simulink model "step_down"  (R2017a)
settings: Solver=VariableStepAuto  StartTime=0  StopTime=1  FixedStep=1e-3  MaxStep=1e-4  RelTol=1e-3
undefined symbols (not defined in the file): C1
libraries: powerlib x71, simulink x3, commsynccomp2 x2, simulink_extras x2, powerlib_meascontrol x2, dsparch4 x1
settings Model: Creator=Bilal Ahmed  LastModifiedBy=Bilal Ahmed

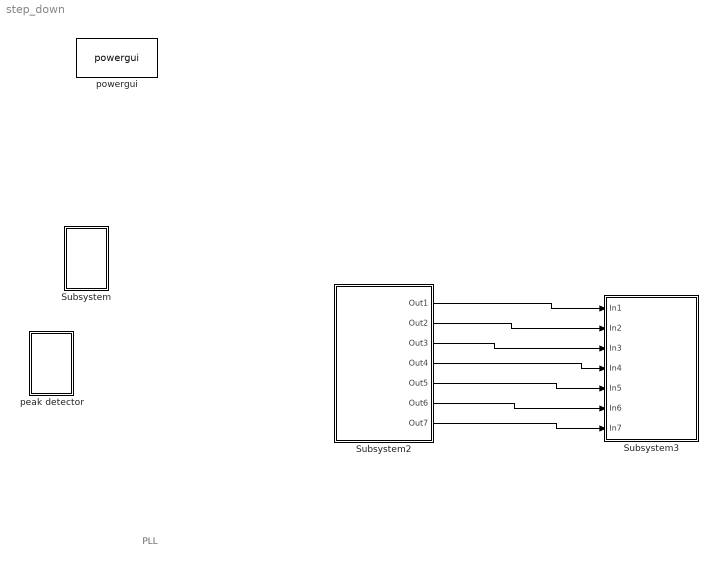
== system step_down ==
  note: PLL
  Subsystem : Subsystem
  Subsystem2 : Subsystem
  Subsystem3 : Subsystem
  peak detector : Subsystem
  powergui : powerlib/powergui  Priority=1  SimulationMode=Continuous  SampleTime=1e-3  frequency=60  Iterations=50  frequencyindice=0  Pbase=100e6  ErrMax=1e-4  UnitsV=kV  UnitsW=MW  buscounter=0  FunctionMessages=off  echomessages=off  EnableUseOfTLC=off  CurrentSourceSwitches=off  DisableSnubberDevices=off  DisableRonSwitches=off  DisableVfSwitches=off  DisplayEquations=off  SolverType=Tustin/Backward Euler (TBE)  Interpol=off  ExternalGateDelay=off  methode=off  Ts=100  x0status=blocks  SPID=on  SwTol=0  HookPort=off  RestoreLinks=warning  ResistiveCurrentMeasurement=off  Frange=[0:2:500]  Ylog=off  Xlog=on  ShowGrid=off  save=off  variable=ZData  structure=0  ZoomFFT=off  StartTime=0.0  cycles=1  DisplayStyle=1  fundamental=60  FreqAxis=off  MaxFrequency=1000  frequencyindicesteady=1  RmsSteady=1  display=off
  wires:
  Subsystem2/1(Out1) -> Subsystem3/1(In1)
  Subsystem2/2(Out2) -> Subsystem3/2(In2)
  Subsystem2/3(Out3) -> Subsystem3/3(In3)
  Subsystem2/4(Out4) -> Subsystem3/4(In4)
  Subsystem2/5(Out5) -> Subsystem3/5(In5)
  Subsystem2/6(Out6) -> Subsystem3/6(In6)
  Subsystem2/7(Out7) -> Subsystem3/7(In7)

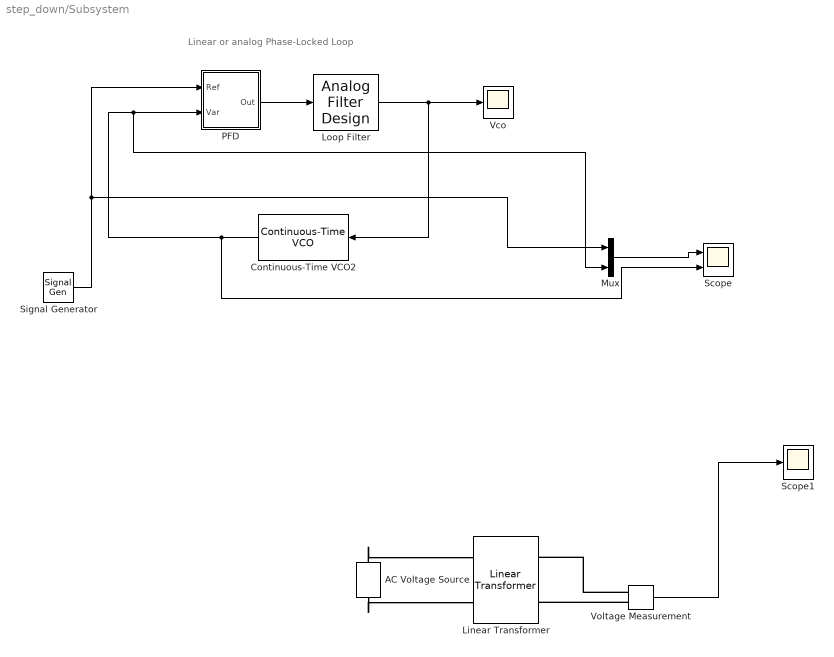
== system step_down/Subsystem ==
  note: Linear or analog Phase-Locked Loop
  AC Voltage Source : powerlib/Electrical Sources/AC Voltage Source  Amplitude=154  Phase=0  Frequency=50  SampleTime=0  Measurements=None  BusType=PV  Pref=10e3  Qref=0  Qmin=-inf  Qmax=+inf
  Continuous-Time VCO2 : commsynccomp2/Continuous-Time VCO  Ac=2  Fc=46  Kc=8  Ph=0
      settings: SourceProductName=Communications System Toolbox  SourceProductBaseCode=CM
  Linear Transformer : powerlib/Elements/Linear Transformer  UNITS=SI  NominalPower=[ 1100 50 ]  winding1=[220 0 0]  winding2=[7 0 0]  ThreeWindings=off  winding3=[3.15e+05 7.8765e+07 26602]  RmLm=[Inf Inf]  Measurements=None  DataType=on
  Loop Filter : dsparch4/Analog Filter Design  method=Butterworth  filttype=Lowpass  N=5  Wlo=50*2*pi  Whi=80  Rp=1  Rs=180
  Mux : Mux  Inputs=2
  PFD : Subsystem
  Scope : Scope  NumInputPorts=2
  Scope1 : Scope
  Signal Generator : SignalGenerator  Amplitude=2  Frequency=2*pi*50  Units=rad/sec
  Vco : Scope
  Voltage Measurement : powerlib/Measurements/Voltage Measurement  PhasorSimulation=off  OutputType=Complex  PSBequivalent=0
  wires:
  Loop Filter/1 -> Vco/1, Continuous-Time VCO2/1
  PFD/1(Out) -> Loop Filter/1
  Mux/1 -> Scope/1
  Continuous-Time VCO2/1 -> Scope/2, Mux/2, PFD/2(Var)
  Signal Generator/1 -> Mux/1, PFD/1(Ref)
  Voltage Measurement/1 -> Scope1/1
  connections:
  AC Voltage Source/RConn1 -- Linear Transformer/LConn1
  AC Voltage Source/LConn1 -- Linear Transformer/LConn2
  Voltage Measurement/LConn1 -- Linear Transformer/RConn1
  Voltage Measurement/LConn2 -- Linear Transformer/RConn2

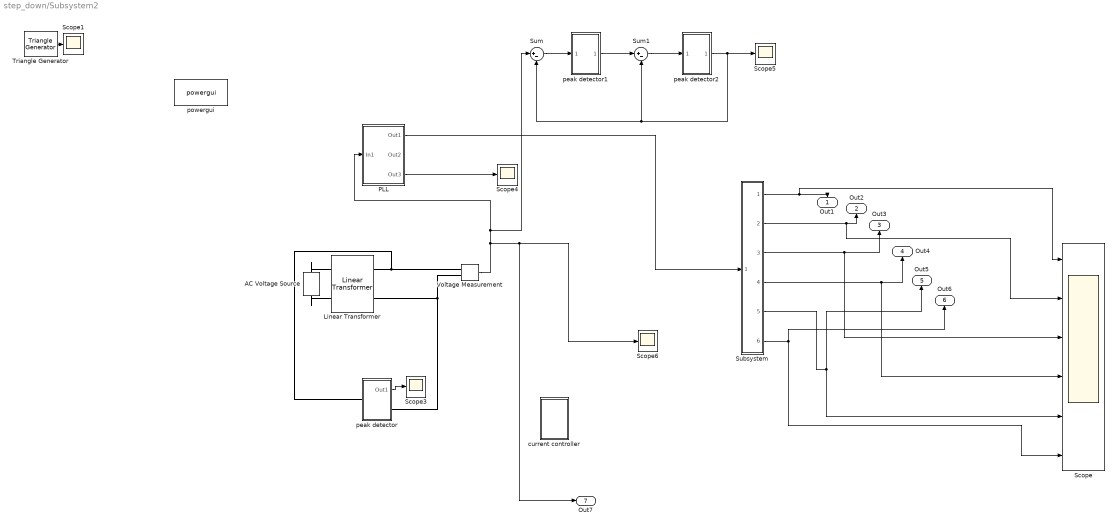
== system step_down/Subsystem2 ==
  AC Voltage Source : powerlib/Electrical Sources/AC Voltage Source  Amplitude=220  Phase=0  Frequency=50  SampleTime=0  Measurements=None  BusType=PV  Pref=10e3  Qref=0  Qmin=-inf  Qmax=+inf
  Linear Transformer : powerlib/Elements/Linear Transformer  UNITS=pu  NominalPower=[1100 50 ]  winding1=[154 0 0]  winding2=[3.5 0 0]  ThreeWindings=off  winding3=[3.15e+05 9.68e-09 3.2267e-07]  RmLm=[Inf Inf]  Measurements=None  DataType=off
  PLL : Subsystem
  Scope : Scope  NumInputPorts=6
  Scope{1,3..6} (5 alike) : Scope
  Subsystem : Subsystem
  Sum : Sum  Inputs=|+-
  Sum1 : Sum  Inputs=|+-
  Triangle Generator : powerlib_meascontrol/Pulse & Signal Generators/Triangle Generator  Freq=1e6  Phase=0  Ts=0
  Voltage Measurement : powerlib/Measurements/Voltage Measurement  PhasorSimulation=off  OutputType=Complex  PSBequivalent=0
  "current controller " : Subsystem
  peak detector : Subsystem
  peak detector1 : Subsystem
  peak detector2 : Subsystem
  powergui : powerlib/powergui  Priority=1  SimulationMode=Continuous  SampleTime=50e-6  frequency=60  Iterations=50  frequencyindice=60  Pbase=100e6  ErrMax=1e-4  UnitsV=kV  UnitsW=MW  buscounter=0  FunctionMessages=off  echomessages=off  EnableUseOfTLC=off  CurrentSourceSwitches=off  DisableSnubberDevices=off  DisableRonSwitches=off  DisableVfSwitches=off  DisplayEquations=off  SolverType=Tustin/Backward Euler (TBE)  Interpol=off  ExternalGateDelay=off  methode=off  Ts=100  x0status=blocks  SPID=on  SwTol=0  HookPort=off  RestoreLinks=warning  ResistiveCurrentMeasurement=off  Frange=[0:2:500]  Ylog=off  Xlog=on  ShowGrid=off  save=off  variable=ZData  structure=0  ZoomFFT=off  StartTime=0.0  cycles=1  DisplayStyle=1  fundamental=60  FreqAxis=off  MaxFrequency=1000  frequencyindicesteady=1  RmsSteady=1  display=off
  Out1 : Outport
  Out2 : Outport  Port=2
  Out3 : Outport  Port=3
  Out4 : Outport  Port=4
  Out5 : Outport  Port=5
  Out6 : Outport  Port=6
  Out7 : Outport  Port=7
  wires:
  Voltage Measurement/1 -> Out7/1, Scope6/1, Sum/1, PLL/1(In1)
  peak detector/1(Out1) -> Scope3/1
  Triangle Generator/1 -> Scope1/1
  PLL/3(Out3) -> Scope4/1
  Subsystem/1(Out1) -> Scope/1, Out1/1
  Subsystem/2(Out2) -> Scope/2, Out2/1
  Subsystem/3(Out3) -> Scope/3, Out3/1
  Subsystem/4(Out4) -> Scope/4, Out4/1
  Subsystem/5(Out5) -> Scope/5, Out5/1
  peak detector1/1(Out1) -> Sum1/1
  peak detector2/1(Out1) -> Sum/2, Sum1/2, Scope5/1
  Sum/1 -> peak detector1/1(In1)
  Sum1/1 -> peak detector2/1(In1)
  Subsystem/6(Out6) -> Scope/6, Out6/1
  PLL/1(Out1) -> Subsystem/1(In1)
  connections:
  Linear Transformer/RConn2 -- peak detector/RConn1 -- Voltage Measurement/LConn2
  AC Voltage Source/LConn1 -- Linear Transformer/LConn2
  Voltage Measurement/LConn1 -- peak detector/LConn1 -- Linear Transformer/RConn1
  AC Voltage Source/RConn1 -- Linear Transformer/LConn1

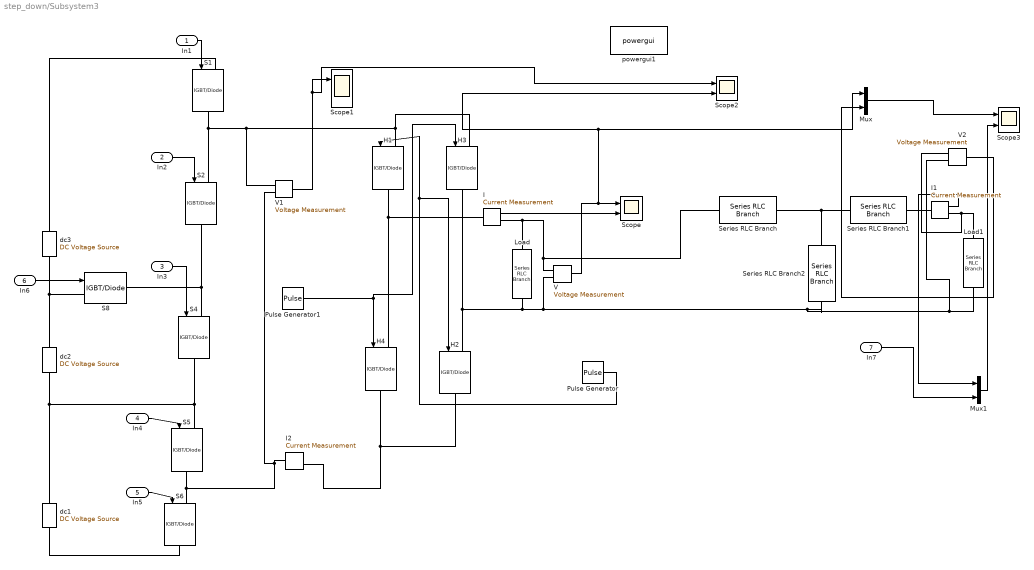
== system step_down/Subsystem3 ==
  In1 : Inport
  In2 : Inport  Port=2
  In3 : Inport  Port=3
  In4 : Inport  Port=4
  In5 : Inport  Port=5
  In6 : Inport  Port=6
  In7 : Inport  Port=7
  H{1..4} (4 alike) : powerlib/Power Electronics/IGBT//Diode  Ron=1e-3  Rs=1e5  Cs=inf  Measurements=off
  I : powerlib/Measurements/Current Measurement  PhasorSimulation=off  OutputType=Complex  PSBequivalent=0
  I1 : powerlib/Measurements/Current Measurement  PhasorSimulation=off  OutputType=Complex  PSBequivalent=0
  I2 : powerlib/Measurements/Current Measurement  PhasorSimulation=off  OutputType=Complex  PSBequivalent=0
  Load : powerlib/Elements/Series RLC Branch  LConnTagsString=__new0  RConnTagsString=__new0  BranchType=R  Resistance=10  Inductance=1e-3  SetiL0=off  InitialCurrent=0  Capacitance=1e-6  Setx0=off  InitialVoltage=0  Measurements=None
  Load1 : powerlib/Elements/Series RLC Branch  LConnTagsString=__new0  RConnTagsString=__new0  BranchType=R  Resistance=10  Inductance=1e-3  SetiL0=off  InitialCurrent=0  Capacitance=1e-6  Setx0=off  InitialVoltage=0  Measurements=None
  Mux : Mux  Inputs=2
  Mux1 : Mux  Inputs=2
  Pulse Generator : DiscretePulseGenerator  PulseType=Time based  Period=0.02  PulseWidth=50
  Pulse Generator1 : DiscretePulseGenerator  PulseType=Time based  Period=0.02  PulseWidth=50  PhaseDelay=.01
  S{1..2,4..6,8} (6 alike) : powerlib/Power Electronics/IGBT//Diode  Ron=1e-3  Rs=1e5  Cs=inf  Measurements=off
  Scope{,1..3} (4 alike) : Scope  NumInputPorts=2
  Series RLC Branch : powerlib/Elements/Series RLC Branch  LConnTagsString=__new0  RConnTagsString=__new0  BranchType=L  Resistance=1  Inductance=1e-3  SetiL0=off  InitialCurrent=0  Capacitance=1e-6  Setx0=off  InitialVoltage=0  Measurements=None
  Series RLC Branch1 : powerlib/Elements/Series RLC Branch  LConnTagsString=__new0  RConnTagsString=__new0  BranchType=L  Resistance=1  Inductance=1e-3  SetiL0=off  InitialCurrent=0  Capacitance=1e-6  Setx0=off  InitialVoltage=0  Measurements=None
  Series RLC Branch2 : powerlib/Elements/Series RLC Branch  LConnTagsString=__new0  RConnTagsString=__new0  BranchType=C  Resistance=1  Inductance=1e-3  SetiL0=off  InitialCurrent=0  Capacitance=1e-6  Setx0=off  InitialVoltage=0  Measurements=None
  V : powerlib/Measurements/Voltage Measurement  PhasorSimulation=off  OutputType=Complex  PSBequivalent=0
  V1 : powerlib/Measurements/Voltage Measurement  PhasorSimulation=off  OutputType=Complex  PSBequivalent=0
  V2 : powerlib/Measurements/Voltage Measurement  PhasorSimulation=off  OutputType=Complex  PSBequivalent=0
  dc1 : powerlib/Electrical Sources/DC Voltage Source  Amplitude=20  Measurements=None
  dc2 : powerlib/Electrical Sources/DC Voltage Source  Amplitude=20  Measurements=None
  dc3 : powerlib/Electrical Sources/DC Voltage Source  Amplitude=20  Measurements=None
  powergui1 : powerlib/powergui  Priority=1  SimulationMode=Continuous  SampleTime=1e-3  frequency=60  Iterations=50  frequencyindice=0  Pbase=100e6  ErrMax=1e-4  UnitsV=kV  UnitsW=MW  buscounter=0  FunctionMessages=off  echomessages=off  EnableUseOfTLC=off  CurrentSourceSwitches=off  DisableSnubberDevices=off  DisableRonSwitches=off  DisableVfSwitches=off  DisplayEquations=off  SolverType=Tustin/Backward Euler (TBE)  Interpol=off  ExternalGateDelay=off  methode=off  Ts=100  x0status=blocks  SPID=on  SwTol=0  HookPort=off  RestoreLinks=warning  ResistiveCurrentMeasurement=off  Frange=[0:2:500]  Ylog=off  Xlog=on  ShowGrid=off  save=off  variable=ZData  structure=0  ZoomFFT=off  StartTime=0.0  cycles=1  DisplayStyle=1  fundamental=60  FreqAxis=off  MaxFrequency=1000  frequencyindicesteady=1  RmsSteady=1  display=off
  wires:
  In3/1 -> S4/1
  In6/1 -> S8/1
  In4/1 -> S5/1
  Pulse Generator1/1 -> H4/1, H3/1
  V/1 -> Mux/1, Scope2/2, Scope/1
  I/1 -> Scope/2
  Pulse Generator/1 -> H1/1, H2/1
  In2/1 -> S2/1
  In1/1 -> S1/1
  In5/1 -> S6/1
  V1/1 -> Scope2/1, Scope1/1
  I1/1 -> Mux1/1
  V2/1 -> Mux/2
  Mux/1 -> Scope3/1
  In7/1 -> Mux1/2
  Mux1/1 -> Scope3/2
  connections:
  H2/RConn1 -- I2/RConn1 -- H4/RConn1
  S2/RConn1 -- S8/RConn1 -- S4/LConn1
  dc2/LConn1 -- S4/RConn1 -- S5/LConn1 -- dc1/RConn1
  dc1/LConn1 -- S6/RConn1
  I/LConn1 -- H4/LConn1 -- H1/RConn1
  H1/LConn1 -- S1/RConn1 -- S2/LConn1 -- V1/LConn1 -- H3/LConn1
  S8/LConn1 -- dc2/RConn1 -- dc3/LConn1
  H2/LConn1 -- H3/RConn1 -- Load/RConn1 -- V2/LConn2 -- Load1/RConn1 -- Series RLC Branch2/RConn1 -- V/LConn2
  dc3/RConn1 -- S1/LConn1
  Load/LConn1 -- I/RConn1 -- Series RLC Branch/LConn1 -- V/LConn1
  S5/RConn1 -- S6/LConn1 -- V1/LConn2 -- I2/LConn1
  Series RLC Branch1/LConn1 -- Series RLC Branch2/LConn1 -- Series RLC Branch/RConn1
  I1/LConn1 -- Series RLC Branch1/RConn1
  I1/RConn1 -- V2/LConn1 -- Load1/LConn1

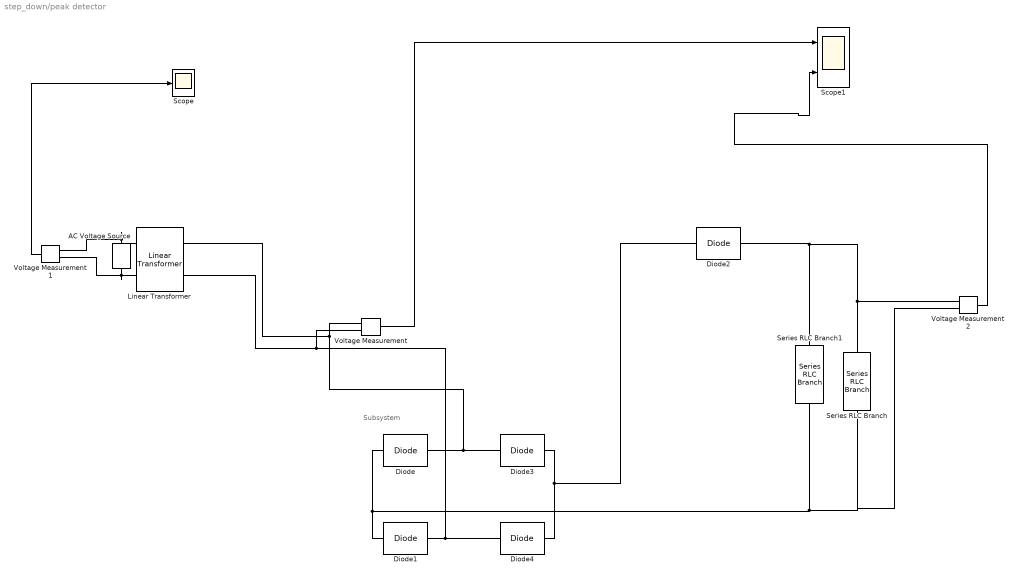
== system step_down/peak detector ==
  note: Subsystem
  AC Voltage Source : powerlib/Electrical Sources/AC Voltage Source  Amplitude=220  Phase=0  Frequency=50  SampleTime=0  Measurements=None  BusType=PV  Pref=10e3  Qref=0  Qmin=-inf  Qmax=+inf
  Diode{,1..4} (5 alike) : powerlib/Power Electronics/Diode  Ron=0.001  Lon=0  Vf=0.03  IC=0  UseSnubber=0  Rs=500  Cs=250e-9  Measurements=off
  Linear Transformer : powerlib/Elements/Linear Transformer  UNITS=SI  NominalPower=[ 1100 50 ]  winding1=[380 0 0]  winding2=[8.641 0 0]  ThreeWindings=off  winding3=[3.15e+05 7.8765e+07 26602]  RmLm=[Inf Inf]  Measurements=None  DataType=on
  Scope : Scope
  Scope1 : Scope  NumInputPorts=2
  Series RLC Branch : powerlib/Elements/Series RLC Branch  LConnTagsString=__new0  RConnTagsString=__new0  BranchType=R  Resistance=1  Inductance=1e-3  SetiL0=off  InitialCurrent=0  Capacitance=1e-6  Setx0=off  InitialVoltage=0  Measurements=None
  Series RLC Branch1 : powerlib/Elements/Series RLC Branch  LConnTagsString=__new0  RConnTagsString=__new0  BranchType=C  Resistance=1  Inductance=1e-3  SetiL0=off  InitialCurrent=0  Capacitance=0.1  Setx0=off  InitialVoltage=0  Measurements=None
  Voltage Measurement : powerlib/Measurements/Voltage Measurement  PhasorSimulation=off  OutputType=Complex  PSBequivalent=0
  Voltage Measurement1 : powerlib/Measurements/Voltage Measurement  PhasorSimulation=off  OutputType=Complex  PSBequivalent=0
  Voltage Measurement2 : powerlib/Measurements/Voltage Measurement  PhasorSimulation=off  OutputType=Complex  PSBequivalent=0
  wires:
  Voltage Measurement1/1 -> Scope/1
  Voltage Measurement/1 -> Scope1/1
  Voltage Measurement2/1 -> Scope1/2
  connections:
  AC Voltage Source/RConn1 -- Voltage Measurement1/LConn1 -- Linear Transformer/LConn1
  AC Voltage Source/LConn1 -- Voltage Measurement1/LConn2 -- Linear Transformer/LConn2
  Diode1/RConn1 -- Diode4/LConn1 -- Linear Transformer/RConn2 -- Voltage Measurement/LConn2
  Diode4/RConn1 -- Diode2/LConn1 -- Diode3/RConn1
  Voltage Measurement/LConn1 -- Linear Transformer/RConn1 -- Diode/RConn1 -- Diode3/LConn1
  Series RLC Branch/RConn1 -- Series RLC Branch1/LConn1 -- Diode2/RConn1 -- Voltage Measurement2/LConn1
  Diode/LConn1 -- Voltage Measurement2/LConn2 -- Series RLC Branch/LConn1 -- Series RLC Branch1/RConn1 -- Diode1/LConn1

== system step_down/Subsystem/PFD ==
  Ref : Inport
  Var : Inport  Port=2
  Product : Product  RndMeth=Zero
  Out : Outport
  wires:
  Ref/1 -> Product/1
  Var/1 -> Product/2
  Product/1 -> Out/1

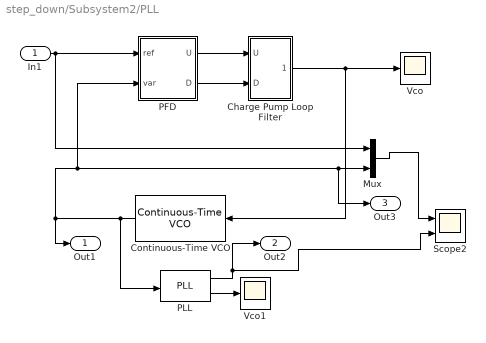
== system step_down/Subsystem2/PLL ==
  In1 : Inport
  Charge Pump Loop Filter : Subsystem
  Continuous-Time VCO : commsynccomp2/Continuous-Time VCO  Ac=5  Fc=45  Kc=3.8  Ph=0
      settings: SourceProductName=Communications System Toolbox  SourceProductBaseCode=CM
  Mux : Mux  Inputs=2
  PFD : Subsystem
  PLL : powerlib_meascontrol/PLL/PLL  Fmin=45  Par_Init=[0, 60]  ParK=[180, 3200, 1]  TcD=1e-4  MaxRateChangeFreq=12  FilterCutOffFreq=25  Ts=0  AGC=on
      settings: SourceProductName=Simscape Power Systems  SourceProductBaseCode=PS
  Scope2 : Scope  NumInputPorts=2
  Vco : Scope
  Vco1 : Scope
  Out1 : Outport
  Out2 : Outport  Port=2
  Out3 : Outport  Port=3
  wires:
  PFD/2(D) -> Charge Pump Loop Filter/2(D)
  In1/1 -> Mux/1, PFD/1(ref)
  Charge Pump Loop Filter/1(contrl) -> Continuous-Time VCO/1, Vco/1
  PFD/1(U) -> Charge Pump Loop Filter/1(U)
  Mux/1 -> Scope2/1
  Continuous-Time VCO/1 -> PLL/1, Out1/1, PFD/2(var), Out3/1, Mux/2
  PLL/1 -> Out2/1, Scope2/2
  PLL/2 -> Vco1/1

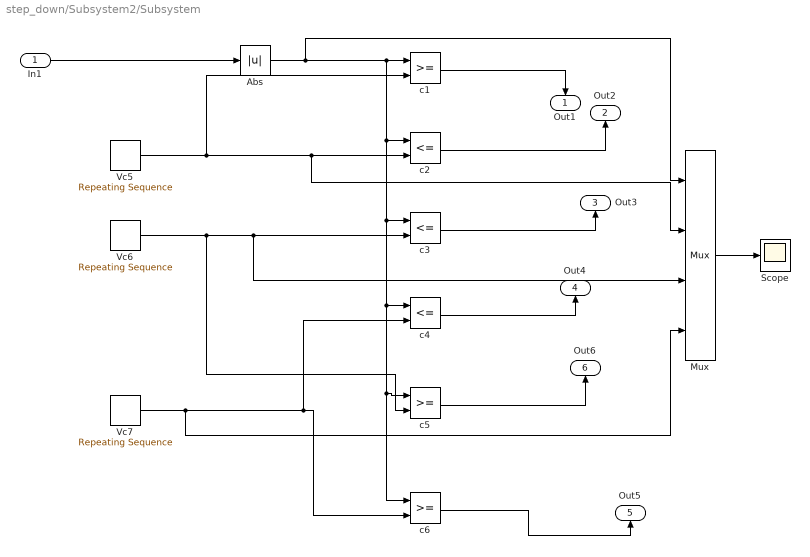
== system step_down/Subsystem2/Subsystem ==
  In1 : Inport
  Abs : Abs
  Mux : Mux
  Scope : Scope
  Vc5 : simulink/Sources/Repeating Sequence  rep_seq_t=[0 0.00001/2 0.00001]  rep_seq_y=[3.3333334 5.0000001 3.3333334]
  Vc6 : simulink/Sources/Repeating Sequence  rep_seq_t=[0 0.00001/2 0.00001]  rep_seq_y=[1.6666667 3.3333334 1.6666667]
  Vc7 : simulink/Sources/Repeating Sequence  rep_seq_t=[0 0.00001/2 0.00001]  rep_seq_y=[0 1.6666667 0]
  c1 : RelationalOperator  OutDataTypeStr=boolean  RndMeth=Nearest
  c2 : RelationalOperator  Operator=<=  OutDataTypeStr=boolean  RndMeth=Nearest
  c3 : RelationalOperator  Operator=<=  OutDataTypeStr=boolean  RndMeth=Nearest
  c4 : RelationalOperator  Operator=<=  OutDataTypeStr=boolean  RndMeth=Nearest
  c5 : RelationalOperator  OutDataTypeStr=boolean  RndMeth=Nearest
  c6 : RelationalOperator  OutDataTypeStr=boolean  RndMeth=Nearest
  Out1 : Outport
  Out2 : Outport  Port=2
  Out3 : Outport  Port=3
  Out4 : Outport  Port=4
  Out5 : Outport  Port=5
  Out6 : Outport  Port=6
  wires:
  c5/1 -> Out6/1
  c6/1 -> Out5/1
  c4/1 -> Out4/1
  c2/1 -> Out2/1
  c1/1 -> Out1/1
  Vc7/1 -> Mux/4, c4/2, c6/2
  Vc5/1 -> c1/2, Mux/2, c2/2
  Vc6/1 -> c5/2, Mux/3, c3/2
  Mux/1 -> Scope/1
  c3/1 -> Out3/1
  Abs/1 -> Mux/1, c2/1, c5/1, c6/1, c4/1, c3/1, c1/1
  In1/1 -> Abs/1

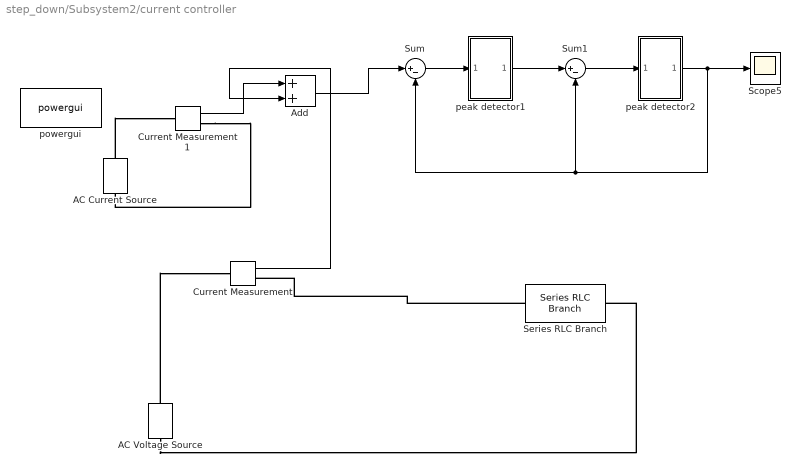
== system step_down/Subsystem2/current controller  ==
  AC Current Source : powerlib/Electrical Sources/AC Current Source  Amplitude=5  Phase=0  Frequency=50  SampleTime=0  Measurements=None
      settings: SourceProductName=Simscape Power Systems  SourceProductBaseCode=PS
  AC Voltage Source : powerlib/Electrical Sources/AC Voltage Source  Amplitude=220  Phase=0  Frequency=20  SampleTime=0  Measurements=None  BusType=swing  Pref=10e3  Qref=0  Qmin=-inf  Qmax=+inf
  Add : Sum
  Current Measurement : powerlib/Measurements/Current Measurement  PhasorSimulation=off  OutputType=Complex  PSBequivalent=0
  Current Measurement1 : powerlib/Measurements/Current Measurement  PhasorSimulation=off  OutputType=Complex  PSBequivalent=0
  Scope5 : Scope
  Series RLC Branch : powerlib/Elements/Series RLC Branch  LConnTagsString=__new0  RConnTagsString=__new0  BranchType=R  Resistance=0.1  Inductance=1e-3  SetiL0=off  InitialCurrent=0  Capacitance=1e-6  Setx0=off  InitialVoltage=0  Measurements=None
  Sum : Sum  Inputs=|+-
  Sum1 : Sum  Inputs=|+-
  peak detector1 : Subsystem
  peak detector2 : Subsystem
  powergui : powerlib/powergui  Priority=1  SimulationMode=Continuous  SampleTime=50e-6  frequency=60  Iterations=50  frequencyindice=20  Pbase=100e6  ErrMax=1e-4  UnitsV=kV  UnitsW=MW  buscounter=0  FunctionMessages=off  echomessages=off  EnableUseOfTLC=off  CurrentSourceSwitches=off  DisableSnubberDevices=off  DisableRonSwitches=off  DisableVfSwitches=off  DisplayEquations=off  SolverType=Tustin/Backward Euler (TBE)  Interpol=off  ExternalGateDelay=off  methode=off  Ts=100  x0status=blocks  SPID=on  SwTol=0  HookPort=off  RestoreLinks=warning  ResistiveCurrentMeasurement=off  Frange=[0:2:500]  Ylog=off  Xlog=on  ShowGrid=off  save=off  variable=ZData  structure=0  ZoomFFT=off  StartTime=0.0  cycles=1  DisplayStyle=1  fundamental=60  FreqAxis=off  MaxFrequency=1000  frequencyindicesteady=1  RmsSteady=1  display=off
  wires:
  peak detector2/1(Out1) -> Sum/2, Sum1/2, Scope5/1
  Sum/1 -> peak detector1/1(In1)
  Sum1/1 -> peak detector2/1(In1)
  peak detector1/1(Out1) -> Sum1/1
  Current Measurement/1 -> Add/2
  Add/1 -> Sum/1
  Current Measurement1/1 -> Add/1
  connections:
  Series RLC Branch/LConn1 -- Current Measurement/RConn1
  AC Voltage Source/RConn1 -- Current Measurement/LConn1
  AC Voltage Source/LConn1 -- Series RLC Branch/RConn1
  Current Measurement1/RConn1 -- AC Current Source/LConn1
  AC Current Source/RConn1 -- Current Measurement1/LConn1

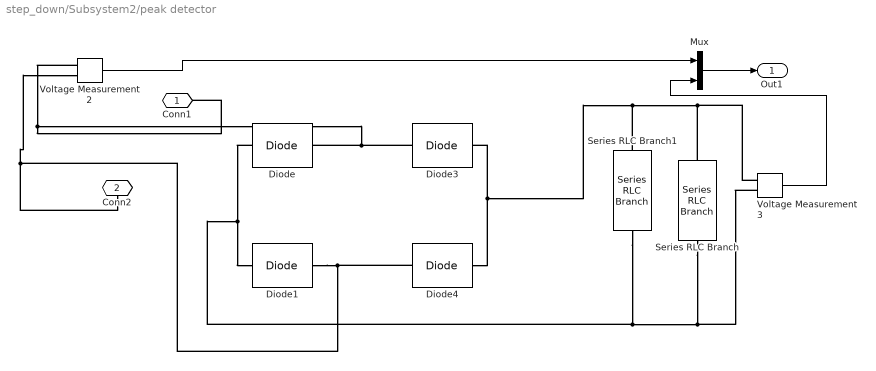
== system step_down/Subsystem2/peak detector ==
  Diode{,1,3..4} (4 alike) : powerlib/Power Electronics/Diode  Ron=0.001  Lon=0  Vf=0.03  IC=0  UseSnubber=0  Rs=500  Cs=250e-9  Measurements=off
  Mux : Mux  Inputs=2
  Series RLC Branch : powerlib/Elements/Series RLC Branch  LConnTagsString=__new0  RConnTagsString=__new0  BranchType=R  Resistance=1  Inductance=1e-3  SetiL0=off  InitialCurrent=0  Capacitance=1e-6  Setx0=off  InitialVoltage=0  Measurements=None
  Series RLC Branch1 : powerlib/Elements/Series RLC Branch  LConnTagsString=__new0  RConnTagsString=__new0  BranchType=C  Resistance=1  Inductance=1e-3  SetiL0=off  InitialCurrent=0  Capacitance=1  Setx0=off  InitialVoltage=0  Measurements=None
  Voltage Measurement2 : powerlib/Measurements/Voltage Measurement  PhasorSimulation=off  OutputType=Complex  PSBequivalent=0
  Voltage Measurement3 : powerlib/Measurements/Voltage Measurement  PhasorSimulation=off  OutputType=Complex  PSBequivalent=0
  Conn1 : PMIOPort  Port=1  Side=Left
  Conn2 : PMIOPort  Port=2  Side=Right
  Out1 : Outport
  wires:
  Voltage Measurement3/1 -> Mux/2
  Voltage Measurement2/1 -> Mux/1
  Mux/1 -> Out1/1
  connections:
  Diode1/RConn1 -- Diode4/LConn1 -- Voltage Measurement2/LConn2 -- Conn2/RConn1
  Diode/LConn1 -- Diode1/LConn1 -- Voltage Measurement3/LConn2 -- Series RLC Branch/LConn1 -- Series RLC Branch1/RConn1
  Diode4/RConn1 -- Diode3/RConn1 -- Voltage Measurement3/LConn1 -- Series RLC Branch/RConn1 -- Series RLC Branch1/LConn1
  Diode/RConn1 -- Voltage Measurement2/LConn1 -- Conn1/RConn1 -- Diode3/LConn1

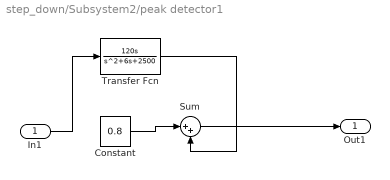
== system step_down/Subsystem2/peak detector1 ==
  In1 : Inport
  Constant : Constant  Value=0.8
  Sum : Sum  Inputs=|++
  Transfer Fcn : TransferFcn  Numerator=[120 0]  Denominator=[1 6 2500]
  Out1 : Outport
  wires:
  In1/1 -> Transfer Fcn/1
  Constant/1 -> Sum/1
  Transfer Fcn/1 -> Sum/2
  Sum/1 -> Out1/1

== system step_down/Subsystem2/peak detector2 ==
  In1 : Inport
  Transfer Fcn1 : TransferFcn  Numerator=[0.013464 1]  Denominator=[0.00462825 0.0380358 2.825 0]
  Out1 : Outport
  wires:
  In1/1 -> Transfer Fcn1/1
  Transfer Fcn1/1 -> Out1/1

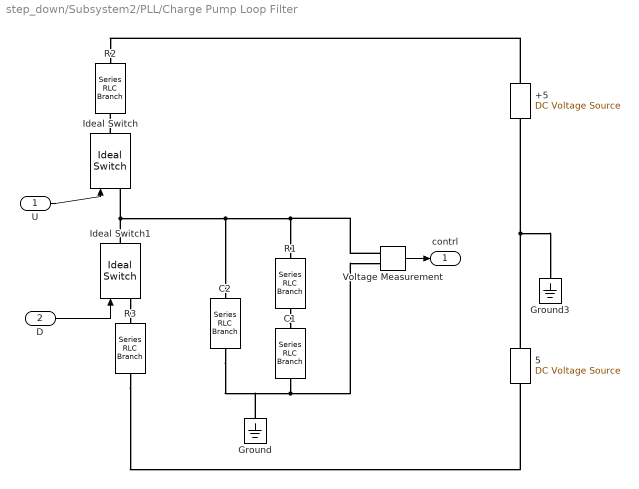
== system step_down/Subsystem2/PLL/Charge Pump Loop Filter ==
  U : Inport
  D : Inport  Port=2
  +5 : powerlib/Electrical Sources/DC Voltage Source  Amplitude=5  Measurements=None
  5 : powerlib/Electrical Sources/DC Voltage Source  Amplitude=5  Measurements=None
  C1 : powerlib/Elements/Series RLC Branch  LConnTagsString=__new0  RConnTagsString=__new0  BranchType=C  Resistance=1  Inductance=1e-3  SetiL0=off  InitialCurrent=0  Capacitance=82e-12  Setx0=off  InitialVoltage=0  Measurements=None
  C2 : powerlib/Elements/Series RLC Branch  LConnTagsString=__new0  RConnTagsString=__new0  BranchType=C  Resistance=1  Inductance=1e-3  SetiL0=off  InitialCurrent=0  Capacitance=17e-12  Setx0=off  InitialVoltage=0  Measurements=None
  Ground : powerlib/Elements/Ground  LConnTagsString=a
  Ground3 : powerlib/Elements/Ground  LConnTagsString=a
  Ideal Switch : powerlib/Power Electronics/Ideal Switch  Ron=0.001  Lon=0  IC=0  Rs=1e8  Cs=inf  Measurements=off
  Ideal Switch1 : powerlib/Power Electronics/Ideal Switch  Ron=0.001  Lon=0  IC=0  Rs=1e8  Cs=inf  Measurements=off
  R1 : powerlib/Elements/Series RLC Branch  LConnTagsString=__new0  RConnTagsString=__new0  BranchType=R  Resistance=11e3  Inductance=1e-3  SetiL0=off  InitialCurrent=0  Capacitance=C1  Setx0=off  InitialVoltage=0  Measurements=None
  R2 : powerlib/Elements/Series RLC Branch  LConnTagsString=__new0  RConnTagsString=__new0  BranchType=R  Resistance=20e3  Inductance=1e-3  SetiL0=off  InitialCurrent=0  Capacitance=C1  Setx0=off  InitialVoltage=0  Measurements=None
  R3 : powerlib/Elements/Series RLC Branch  LConnTagsString=__new0  RConnTagsString=__new0  BranchType=R  Resistance=20e3  Inductance=1e-3  SetiL0=off  InitialCurrent=0  Capacitance=C1  Setx0=off  InitialVoltage=0  Measurements=None
  Voltage Measurement : powerlib/Measurements/Voltage Measurement  PhasorSimulation=off  OutputType=Complex  PSBequivalent=0
  contrl : Outport
  wires:
  D/1 -> Ideal Switch1/1
  Voltage Measurement/1 -> contrl/1
  U/1 -> Ideal Switch/1
  connections:
  R1/RConn1 -- C1/LConn1
  C1/RConn1 -- Ground/LConn1 -- C2/RConn1 -- Voltage Measurement/LConn2
  Ideal Switch1/RConn1 -- C2/LConn1 -- R1/LConn1 -- Voltage Measurement/LConn1 -- Ideal Switch/LConn1
  R3/RConn1 -- 5/LConn1
  Ideal Switch1/LConn1 -- R3/LConn1
  Ideal Switch/RConn1 -- R2/RConn1
  5/RConn1 -- +5/LConn1 -- Ground3/LConn1
  +5/RConn1 -- R2/LConn1

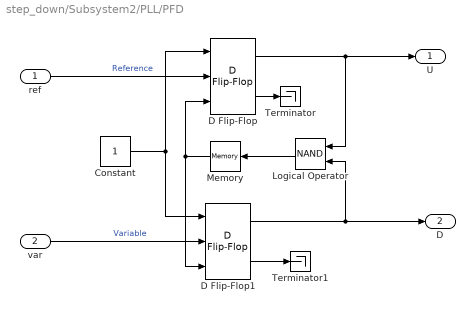
== system step_down/Subsystem2/PLL/PFD ==
  ref : Inport
  var : Inport  Port=2
  Constant : Constant  OutDataTypeStr=boolean
  D Flip-Flop : simulink_extras/Flip Flops/D Flip-Flop
      settings: SourceProductName=Simulink
  D Flip-Flop1 : simulink_extras/Flip Flops/D Flip-Flop
      settings: SourceProductName=Simulink
  Logical Operator : Logic  Operator=NAND
  Memory : Memory
  Terminator : Terminator
  Terminator1 : Terminator
  U : Outport
  D : Outport  Port=2
  wires:
  D Flip-Flop/2 -> Terminator/1
  D Flip-Flop1/2 -> Terminator1/1
  Logical Operator/1 -> Memory/1
  ref/1 -> D Flip-Flop/2  "Reference"
  var/1 -> D Flip-Flop1/2  "Variable"
  Constant/1 -> D Flip-Flop/1, D Flip-Flop1/1
  Memory/1 -> D Flip-Flop/3, D Flip-Flop1/3
  D Flip-Flop/1 -> U/1, Logical Operator/1
  D Flip-Flop1/1 -> D/1, Logical Operator/2

== system step_down/Subsystem2/current controller /peak detector1 ==
  In1 : Inport
  Transfer Fcn : TransferFcn  Numerator=[0.8 124.8 2000]  Denominator=[1 6 2500]
  Out1 : Outport
  wires:
  In1/1 -> Transfer Fcn/1
  Transfer Fcn/1 -> Out1/1

== system step_down/Subsystem2/current controller /peak detector2 ==
  In1 : Inport
  Transfer Fcn1 : TransferFcn  Numerator=[0.013464 1]  Denominator=[0.00462825 0.0380358 2.825 0]
  Out1 : Outport
  wires:
  In1/1 -> Transfer Fcn1/1
  Transfer Fcn1/1 -> Out1/1
